simulink model "Constant_cases"  (R2023a)
settings: Solver=VariableStepAuto  StartTime=0.0  StopTime=10  RelTol=1e-3
settings Model: Creator=HP  LastModifiedBy=HP

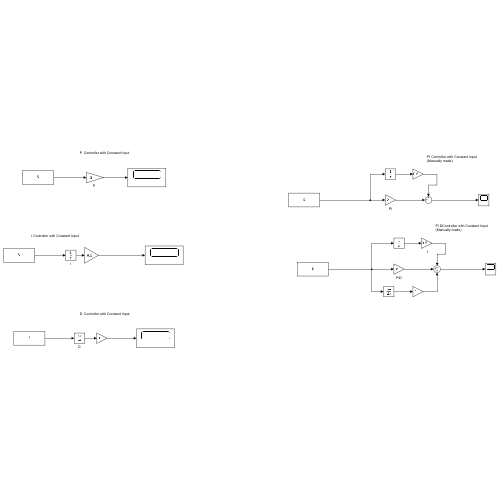
[thumbnail: Simulink's stored preview of the top-level diagram]
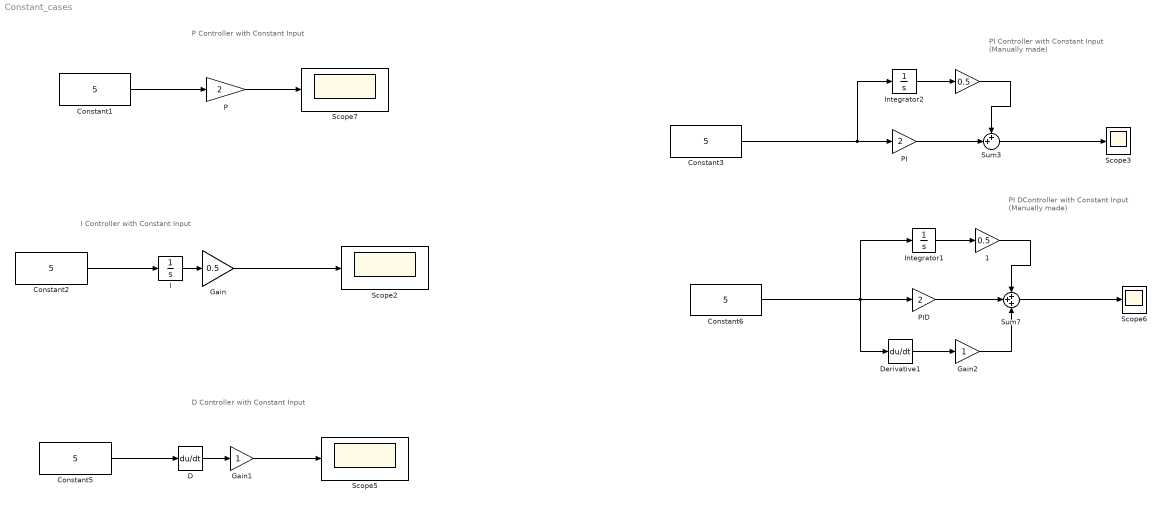
== system Constant_cases ==
  note: I Controller with Constant Input
  note: P Controller with Constant Input
  note: PI Controller with Constant Input
      | (Manually made)
  note: D Controller with Constant Input
  note: PI DController with Constant Input
      | (Manually made)
  " " : Gain  Gain=0.5
  " 1" : Gain  Gain=0.5
  Constant{1..3,5..6} (5 alike) : Constant  Value=5
  D : Derivative
  Derivative1 : Derivative
  Gain : Gain  Gain=0.5
  Gain1 : Gain
  Gain2 : Gain
  I : Integrator
  Integrator1 : Integrator
  Integrator2 : Integrator
  "P  " : Gain  Gain=2
  PI : Gain  Gain=2
  PID : Gain  Gain=2
  Scope{2..3,5..7} (5 alike) : Scope
  Sum3 : Sum  Inputs=++|
  Sum7 : Sum  Inputs=+++
  wires:
  Constant1/1 -> "P  "/1
  " "/1 -> Sum3/1
  PI/1 -> Sum3/2
  Integrator2/1 -> " "/1
  Constant2/1 -> I/1
  I/1 -> Gain/1
  Constant3/1 -> Integrator2/1, PI/1
  D/1 -> Gain1/1
  Constant6/1 -> Derivative1/1, PID/1, Integrator1/1
  PID/1 -> Sum7/2
  " 1"/1 -> Sum7/1
  Integrator1/1 -> " 1"/1
  Derivative1/1 -> Gain2/1
  Gain2/1 -> Sum7/3
  "P  "/1 -> Scope7/1
  Gain1/1 -> Scope5/1
  Gain/1 -> Scope2/1
  Sum3/1 -> Scope3/1
  Sum7/1 -> Scope6/1
  Constant5/1 -> D/1
